simulink model "unitTestAircraftState"  (R2018b)
settings: Solver=VariableStepAuto  StartTime=0.0  StopTime=100  RelTol=1e-3
libraries: AircraftStateFromPositions x1
settings Model: Creator=PE29732  LastModifiedBy=PE29732

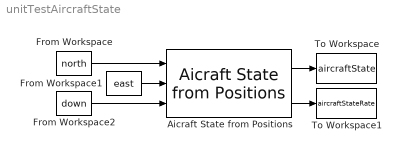
== system unitTestAircraftState ==
  Aicraft State from Positions : AircraftStateFromPositions/Aicraft State from Positions
  From Workspace : FromWorkspace  VariableName=north  SampleTime=0
  From Workspace1 : FromWorkspace  VariableName=east  SampleTime=0
  From Workspace2 : FromWorkspace  VariableName=down  SampleTime=0
  To Workspace : ToWorkspace  VariableName=aircraftState  SaveFormat=Timeseries  SampleTime=-1
  To Workspace1 : ToWorkspace  VariableName=aircraftStateRate  SaveFormat=Timeseries  SampleTime=-1
  wires:
  From Workspace/1 -> Aicraft State from Positions/1
  From Workspace1/1 -> Aicraft State from Positions/2
  From Workspace2/1 -> Aicraft State from Positions/3
  Aicraft State from Positions/1 -> To Workspace/1
  Aicraft State from Positions/2 -> To Workspace1/1
